simulink model "ReachCoreachDemo_v2_2011"  (Simulink 7.8)
settings: Solver=ode45  StartTime=0.0  StopTime=10.0  RelTol=1e-3
settings Model: Creator=T6684MB  LastModifiedBy=gm
settings DebuggingCC: FrameProcessingCompatibilityMsg=error
settings CodeAppCC: CustomSymbolStrType=$N$R$M_T
settings GRTTargetCC: TargetFunctionLibrary=C89/C90 (ANSI)

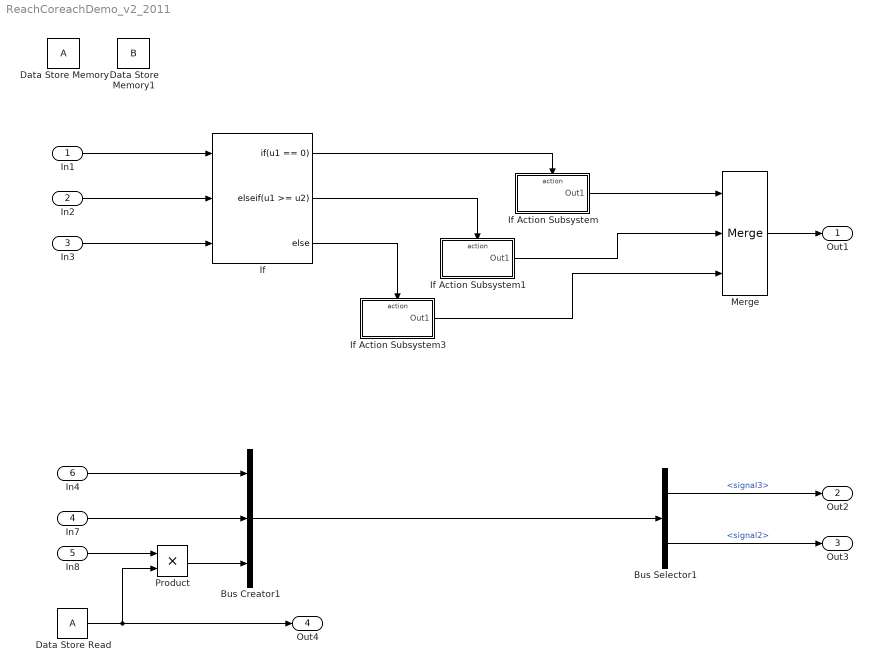
== system ReachCoreachDemo_v2_2011 ==
  In1 : Inport
  In2 : Inport  Port=2
  In3 : Inport  Port=3
  In7 : Inport  Port=4
  In8 : Inport  Port=5
  In4 : Inport  Port=6
  Bus Creator1 : BusCreator  Inputs=3
  Bus Selector1 : BusSelector  OutputSignals=signal3,signal2
  Data Store Memory : DataStoreMemory  ReadBeforeWriteMsg=warning  WriteAfterWriteMsg=warning  WriteAfterReadMsg=warning  ShowAdditionalParam=off
  Data Store Memory1 : DataStoreMemory  DataStoreName=B  ReadBeforeWriteMsg=warning  WriteAfterWriteMsg=warning  WriteAfterReadMsg=warning  ShowAdditionalParam=off
  Data Store Read : DataStoreRead
  If : If  NumInputs=3  IfExpression=u1 == 0  ElseIfExpressions=u1 >= u2
  If Action Subsystem : Subsystem  TreatAsAtomicUnit=on
  If Action Subsystem1 : Subsystem  TreatAsAtomicUnit=on
  If Action Subsystem3 : Subsystem  TreatAsAtomicUnit=on
  Merge : Merge  Inputs=3
  Product : Product
  Out1 : Outport
  Out2 : Outport  Port=2
  Out3 : Outport  Port=3
  Out4 : Outport  Port=4
  wires:
  In1/1 -> If/1
  If/1 -> If Action Subsystem/Action
  If/2 -> If Action Subsystem1/Action
  If/3 -> If Action Subsystem3/Action
  If Action Subsystem/1(Out1) -> Merge/1
  If Action Subsystem1/1(Out1) -> Merge/2
  Merge/1 -> Out1/1
  In2/1 -> If/2
  In3/1 -> If/3
  If Action Subsystem3/1(Out1) -> Merge/3
  Bus Creator1/1 -> Bus Selector1/1
  Bus Selector1/1 -> Out2/1  "<signal3>"
  In8/1 -> Product/1
  Bus Selector1/2 -> Out3/1  "<signal2>"
  Product/1 -> Bus Creator1/3
  In4/1 -> Bus Creator1/1
  In7/1 -> Bus Creator1/2
  Data Store Read/1 -> Out4/1, Product/2

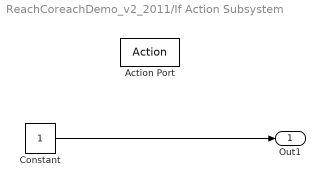
== system ReachCoreachDemo_v2_2011/If Action Subsystem ==
  Action Port : ActionPort
  Constant : Constant
  Out1 : Outport  InitialOutput=1
  wires:
  Constant/1 -> Out1/1

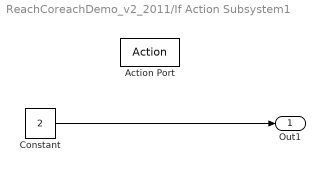
== system ReachCoreachDemo_v2_2011/If Action Subsystem1 ==
  Action Port : ActionPort
  Constant : Constant  Value=2
  Out1 : Outport  InitialOutput=2
  wires:
  Constant/1 -> Out1/1

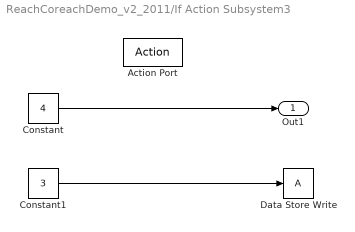
== system ReachCoreachDemo_v2_2011/If Action Subsystem3 ==
  Action Port : ActionPort
  Constant : Constant  Value=4
  Constant1 : Constant  Value=3
  Data Store Write : DataStoreWrite
  Out1 : Outport  InitialOutput=4
  wires:
  Constant/1 -> Out1/1
  Constant1/1 -> Data Store Write/1
